simulink model "LQR_model"  (R2021a)
settings: Solver=FixedStepAuto  StartTime=0.0  StopTime=3  FixedStep=0.01  RelTol=1e-3
settings Model: Creator=Shayan  LastModifiedBy=SHAMBHAVI
settings SolverCC: AlgebraicLoopSolver=TrustRegion
settings DataIOCC: ReturnWorkspaceOutputs=off
settings OptimizationCC: LifeSpan=inf
settings DebuggingCC: SFMachineParentedDataDiag=warning  ArithmeticOperatorsInVariantConditions=warning
settings SFSimCC: CustomCodeUndefinedFunction=UseInterfaceOnly
settings CodeAppCC: StateflowObjectComments=on

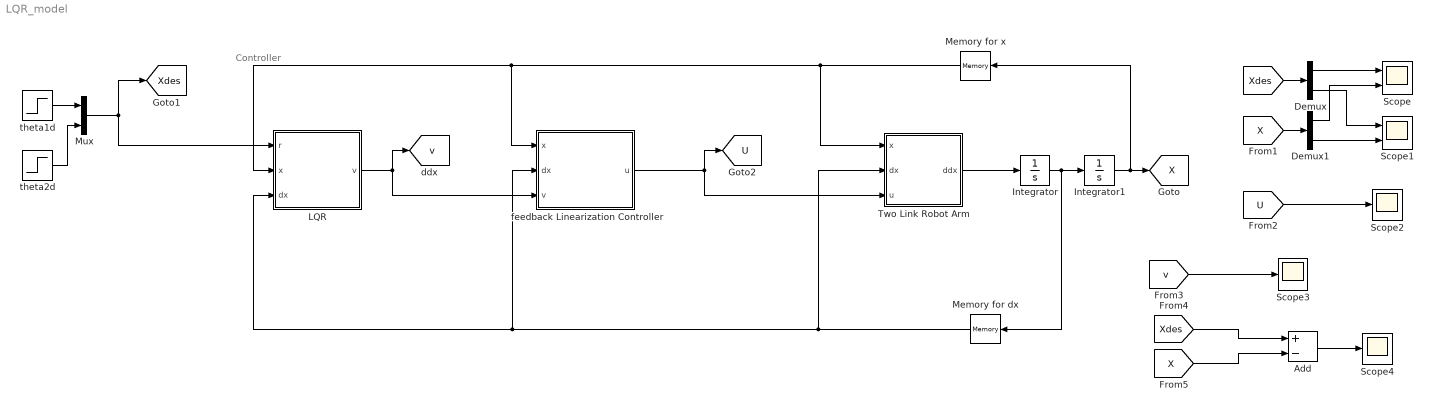
== system LQR_model ==
  note: Controller
  Add : Sum  Inputs=+-
  Demux : Demux  Outputs=2
  Demux1 : Demux  Outputs=2
  Integrator : Integrator  InitialCondition=[0 0]
  Integrator1 : Integrator  InitialCondition=[pi/2 -pi/2]
  LQR : MATLAB Function  TreatAsAtomicUnit=on
  Memory for dx : Memory  InitialCondition=[0 0]
  Memory for x : Memory  InitialCondition=[pi/2 -pi/2]
  Mux : Mux  Inputs=2
  Scope : Scope  NumInputPorts=2
  Scope1 : Scope  NumInputPorts=2
  Scope2 : Scope
  Scope3 : Scope
  Scope4 : Scope
  Two Link Robot Arm : MATLAB Function  TreatAsAtomicUnit=on
  feedback Linearization Controller : MATLAB Function  TreatAsAtomicUnit=on
  theta1d : Step  Time=0  After=-pi/2  SampleTime=0
  theta2d : Step  Time=0  After=pi/2  SampleTime=0
  tag scope: U=global, X=global, Xdes=global, v=global
  wires:
  Integrator/1 -> Memory for dx/1, Integrator1/1
  Two Link Robot Arm/1(ddx) -> Integrator/1
  Integrator1/1 -> [X], Memory for x/1
  theta1d/1 -> Mux/1
  theta2d/1 -> Mux/2
  feedback Linearization Controller/1(u) -> Two Link Robot Arm/3(u), [U]
  [Xdes] -> Demux/1
  [X] -> Demux1/1
  Demux/1 -> Scope/1
  Demux1/1 -> Scope/2
  Demux1/2 -> Scope1/2
  Demux/2 -> Scope1/1
  [U] -> Scope2/1
  [v] -> Scope3/1
  [Xdes] -> Add/1
  [X] -> Add/2
  Add/1 -> Scope4/1
  Memory for dx/1 -> Two Link Robot Arm/2(dx), LQR/3(dx), feedback Linearization Controller/2(dx)
  LQR/1(v) -> feedback Linearization Controller/3(v), [v]
  Memory for x/1 -> Two Link Robot Arm/1(x), LQR/2(x), feedback Linearization Controller/1(x)
  Mux/1 -> LQR/1(r), [Xdes]

== matlab function LQR_model/feedback Linearization Controller ==
  data: x input; dx input; u output; v input
function u = fcn(x,dx,v)

M1 = 1;
M2 = 1;
L1 = 1;
L2 = 1;
g = 9.81;
G = [-(M1+M2)*g*L1-M2*g*L2*sin(x(1)+x(2));...
    -M2*g*L2*sin(x(1)+x(2));]; %gravitational 
C = [M1*L1*L2*(2*dx(1)*dx(2) + dx(1)^2)*sin(x(2));...
    -M2*L1*L2*dx(1)*dx(2)*sin(x(2));]; %coriolis
M = [-(M1+M2)*L1^2 + M2*L2^2 + 2*M2*L1*L2*cos(x(2)), M2*L2^2 + M2*L1*L2*cos(x(2));...
     M2*L2^2 + M2*L1*L2*cos(x(2)),  M2*L2^2;]; %intertial component

u = M*v + C + G; %two dimensional torque vector coloumn matrix

== matlab function LQR_model/Two Link Robot Arm ==
  data: x input; dx input; u input; ddx output
function ddx = fcn(x,dx,u)

M1 = 1;
M2 = 1;
L1 = 1;
L2 = 1;
g = 9.81;
G = [-(M1+M2)*g*L1-M2*g*L2*sin(x(1)+x(2));...
    -M2*g*L2*sin(x(1)+x(2));];
C = [M1*L1*L2*(2*dx(1)*dx(2) + dx(1)^2)*sin(x(2));...
    -M2*L1*L2*dx(1)*dx(2)*sin(x(2));];
M = [-(M1+M2)*L1^2 + M2*L2^2 + 2*M2*L1*L2*cos(x(2)), M2*L2^2 + M2*L1*L2*cos(x(2));...
     M2*L2^2 + M2*L1*L2*cos(x(2)),  M2*L2^2;];
ddx = inv(M)*(-C-G+u);

== matlab function LQR_model/LQR ==
  data: r input; v output; x input; dx input
function v  = fcn(r,x,dx)
%r is the reference angle r(1) = -pi/2 and r(2)=pi/2
%System Dynamics
A=[0    1;
   0    0];
B=[0;
   1];
C=[1 0];
D=0;

%Control Law
%changing Q and R would change weights of performance and effort resp?
Q=[1 0; %Penalise angular error
   0 0]; %Penalise angular rate

R=1; %Penalise thruster effort, positive constant

K=lqr(A,B,Q,R);

%Closed Loop System
sys=ss((A-B*K),B,C,D);

%Run response to initial condition
t=0:0.005:30
[y,t,x]=initial(sys, x0, t);

v=[k1*(r(1)-x(1))+k2*dx(1);...
    k1*(r(2)-x(2))+k2*dx(2);];
